simulink model "valveflow"  (R2020b)
settings: Solver=VariableStepAuto  StartTime=0.0  StopTime=inf  RelTol=1e-3
libraries: opclib x3, sldrtlib x1
settings Model: Creator=Ferdy  LastModifiedBy=Asus

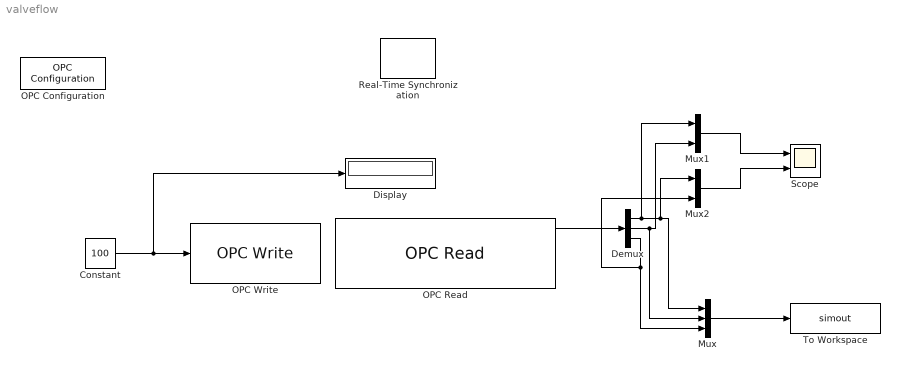
== system valveflow ==
  Constant : Constant  Value=100
  Demux : Demux  Outputs=3
  Display : Display
  Mux : Mux  Inputs=3
  Mux1 : Mux  Inputs=2
  Mux2 : Mux  Inputs=2
  OPC Configuration : opclib/OPC Configuration  opcServers=localhost/KEPware.KEPServerEx.V4/10  errMissingItems=Error  errReadWrite=Warn  errShutdown=Error  errRTViolation=Warn  rtEnable=on  speedup=1  showLatency=off  beingUsed=on
      settings: SourceProductBaseCode=OT
  OPC Read : opclib/OPC Read  serverHost=localhost  serverID=KEPware.KEPServerEx.V4  itemIDs=Fultek.CPU101F.ControlValve, Fultek.CPU101F.InputFlow, Fultek.CPU101F.Output_LPM  readMode=Synchronous (cache)  dataType=double  updateRate=0.5  showQual=on  showTS=on  tsMode=Seconds since start
      settings: SourceProductBaseCode=OT
  OPC Write : opclib/OPC Write  serverHost=localhost  serverID=KEPware.KEPServerEx.V4  itemIDs=Fultek.CPU101F.ControlValve  writeMode=Synchronous  updateRate=0
      settings: SourceProductBaseCode=OT
  Real-Time Synchronization : sldrtlib/Real-Time Synchronization  SampleTime=0.1  MaxMissedTicks=10  ShowMissedTicks=off  YieldWhenWaiting=off
  Scope : Scope  NumInputPorts=2
  To Workspace : ToWorkspace  VariableName=simout  SaveFormat=Timeseries  SampleTime=-1
  wires:
  Constant/1 -> Display/1, OPC Write/1
  OPC Read/1 -> Demux/1
  Mux/1 -> To Workspace/1
  Demux/1 -> Mux1/1, Mux2/1, Mux/1
  Demux/2 -> Mux1/2, Mux/2
  Demux/3 -> Mux2/2, Mux/3
  Mux1/1 -> Scope/1
  Mux2/1 -> Scope/2
